simulink library "LATCH_ERROR_LIB"  (R2021b)
settings: Solver=VariableStepAuto  StartTime=0.0  StopTime=10.0  RelTol=1e-3
settings Model: Creator=C83127  LastModifiedBy=ACH

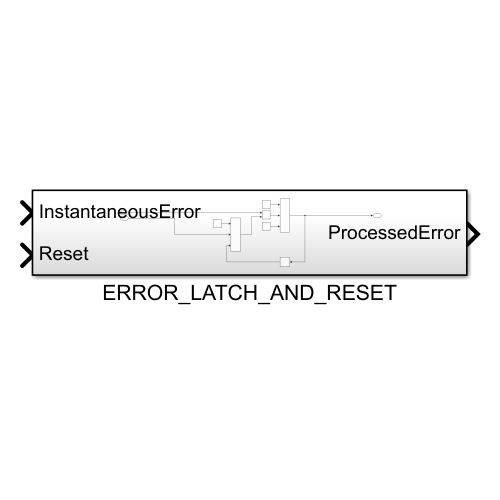
[thumbnail: Simulink's stored preview of the top-level diagram]
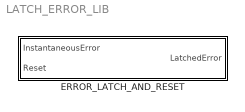
== system LATCH_ERROR_LIB ==
  ERROR_LATCH_AND_RESET : Subsystem

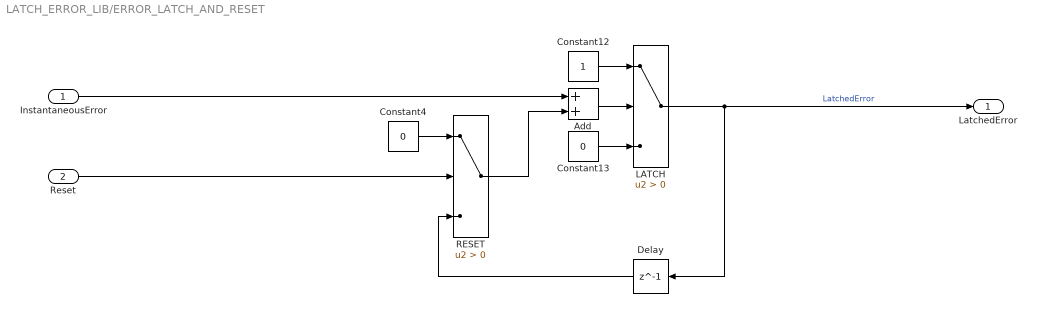
== system LATCH_ERROR_LIB/ERROR_LATCH_AND_RESET ==
  InstantaneousError : Inport
  Reset : Inport  Port=2
  Add : Sum
  Constant12 : Constant
  Constant13 : Constant  Value=0
  Constant4 : Constant  Value=0
  Delay : Delay  DelayLength=1
  LATCH : Switch  Criteria=u2 > Threshold
  RESET : Switch  Criteria=u2 > Threshold
  LatchedError : Outport
  wires:
  LATCH/1 -> LatchedError/1, Delay/1  "LatchedError"
  Constant12/1 -> LATCH/1
  Constant13/1 -> LATCH/3
  Constant4/1 -> RESET/1
  Delay/1 -> RESET/3
  Add/1 -> LATCH/2
  RESET/1 -> Add/2
  InstantaneousError/1 -> Add/1
  Reset/1 -> RESET/2
